simulink model "DrivingTestBench"  (R2026a)
settings: Solver=ode3  StartTime=0  StopTime=30  FixedStep=Ts  MaxStep=Ts
PreLoadFcn:
  | if(~configureDrivingTestBench.isdrivingApplicationOnPath())
  |     pathToDrivingApplication = fullfile(...
  |         matlabshared.supportpkg.getSupportPackageRoot,...
  |         "toolbox", "driving", "supportpackages", "variantgenerator", "drivingApplication");
  | 
  | 
  |     if (~exist("pathToDrivingApplication", "dir"))
  |         sldiagviewer.reportError(['This model requires you to download and install '...
  |             'Automated Driving Toolbox™ Test Suite for Euro NCAP® Protocols']);
  |     else
  |         addpath(fullfile(matlabshared.supportpkg.getSupportPackageRoot,"toolbox", "driving", "supportpackages", "variantgenerator", "drivingApplication"));
  |     end
  | end
values from neighbouring files (symbols this model uses):
  actorProfiles = repmat(actorProfile, 1, numActors)    [configureDrivingTestBench.m]
  BusActorPoses = Simulink.Bus    [configureDrivingTestBench.m]
  egoVehDyn = egoVehicleDynamicsParams(obj, egoInitialPose, actorProfiles(egoIndex))    [configureDrivingTestBench.m]
  m = worldActors(idx).actor_runtime.pose.matrix    [configureDrivingTestBench.m]
  maxAcc = 6    [configureDrivingTestBench.m]
  n = length(i)    [TargetBehavior.m]
  testStartPosition = [egoStartXPos egoStartYPos egoStartZPos]    [configureDrivingTestBench.m]
undefined symbols (not defined in the file or in its folder): aebEnable, cameraParams, Defined, driving, dtleThreshold, Ego, egoActorID, egoPathWidth, Lane, Left, lkaEnable, matlabshared, maxDecel, maxNumActors, Right, steadyStateSpeed, trackingParams, trackPosSelector, Ts, User
libraries: roadrunnerscenario x6, simulink_extras x6, drivingscenarioandsensors x4, trackingutilitieslib x1, drivinglib x1, simulink x1, autolibutils x1, autolibshared x1
(part 1 of 2)
settings Model: SILPILSystemUnderTest=refmodels  PauseTimes=16  SnapshotInterval=5  PacingRate=0.220000  Creator=The MathWorks, Inc.  LastModifiedBy=mraj
settings SolverCC: ZeroCrossAlgorithm=Adaptive  MinimalZcImpactIntegration=on
settings OptimizationCC: InlineInvariantSignals=on  SimCompilerOptimization=on
settings DebuggingCC: BusObjectLabelMismatch=none  PregeneratedLibrarySubsystemCodeDiagnostic=none  SubsystemReferenceDiagnosticForUnitTest=warning
settings ModelReferenceCC: CheckModelReferenceTargetMessage=none  EnableParallelModelReferenceBuilds=on  ModelReferenceNumInstancesAllowed=Single  PropagateVarSize=Only when enabling
settings RTWCC: SystemTargetFile=ert.tlc  GenerateReport=on  BuildConfiguration=Faster Runs  LaunchReport=on  LargeConstantGeneration=WriteOnlyDNNConstantsToDataFiles  Description=Embedded Coder
settings ERTTargetCC: DynamicArrayContainerType=coder::array  GenerateSampleERTMain=on
settings SimscapeCC: SimscapeNominalValues="[{\"value\":\"1\",\"unit\":\"A\"},{\"value\":\"1\",\"unit\":\"bar\"},{\"value\":\"1\",\"unit\":\"cm^2\"},{\"value\":\"1\",\"unit\":\"cm^3/s\"},{\"value\":\"1\",\"unit\":\"kJ/kg\"},{\"value\":\"1\",\"unit\":\"kW\"},{\"value\":\"1\",\"unit\":\"l\"},{\"value\":\"1\",\"unit\":\"N\"},{\"value\":\"1\",\"unit\":\"N*m\"},{\"value\":\"1\",\"unit\":\"V\"}]"  SimscapeLogType=none  SimscapeLogDataHistory=5000.0

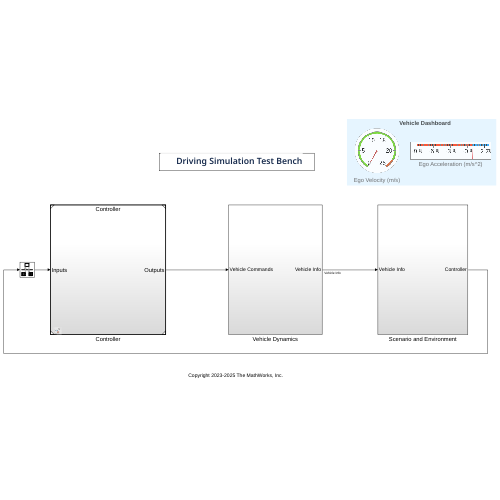
[thumbnail: Simulink's stored preview of the top-level diagram]
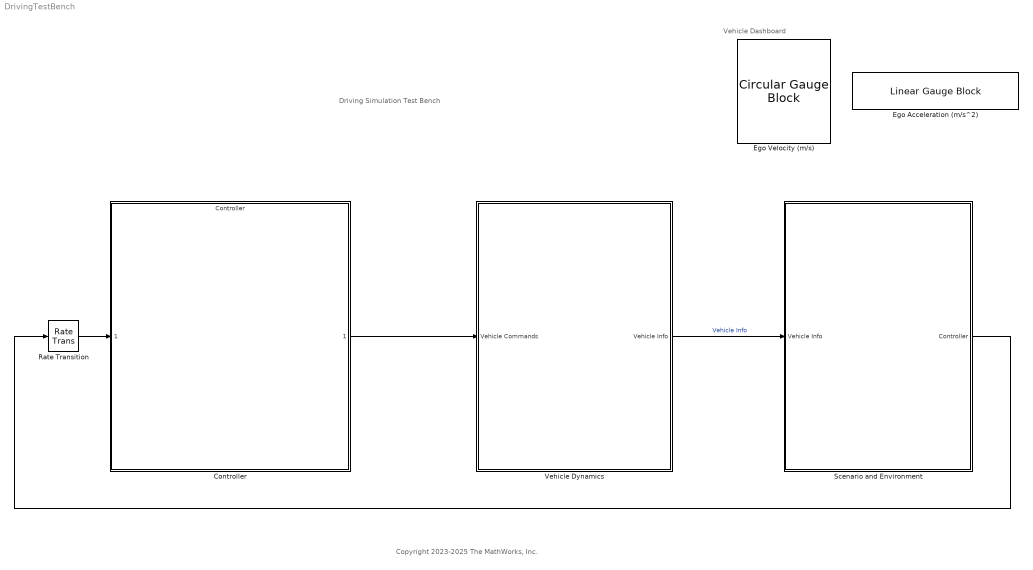
== system DrivingTestBench ==
  note: Copyright 2023-2025 The MathWorks, Inc.
  note: Driving Simulation Test Bench
  note: Vehicle Dashboard
  Controller : ModelReference  ModelNameDialog=Controller.slx  SimulationMode=Normal  CodeInterface=Top model  ModelReferenceVersion=12.11
  Ego Acceleration (m/s^2) : LinearGaugeBlock  LabelPosition=Hide  ScaleMin=-9.8  ScaleMax=3  TickInterval=3  FontColor=[0.0, 0.0, 0.0]
  Ego Velocity (m/s) : CircularGaugeBlock  LabelPosition=Hide  ScaleMax=25  FontColor=[0.0, 0.0, 0.0]
  Rate Transition : RateTransition  OutPortSampleTime=ControllerStepSize
  Scenario and Environment : Subsystem
  Vehicle Dynamics : Subsystem
  wires:
  Vehicle Dynamics/1(Vehicle Info) -> Scenario and Environment/1(Vehicle Info)  "Vehicle Info"
  Controller/1 -> Vehicle Dynamics/1(Vehicle Commands)
  Scenario and Environment/1(Controller) -> Rate Transition/1
  Rate Transition/1 -> Controller/1

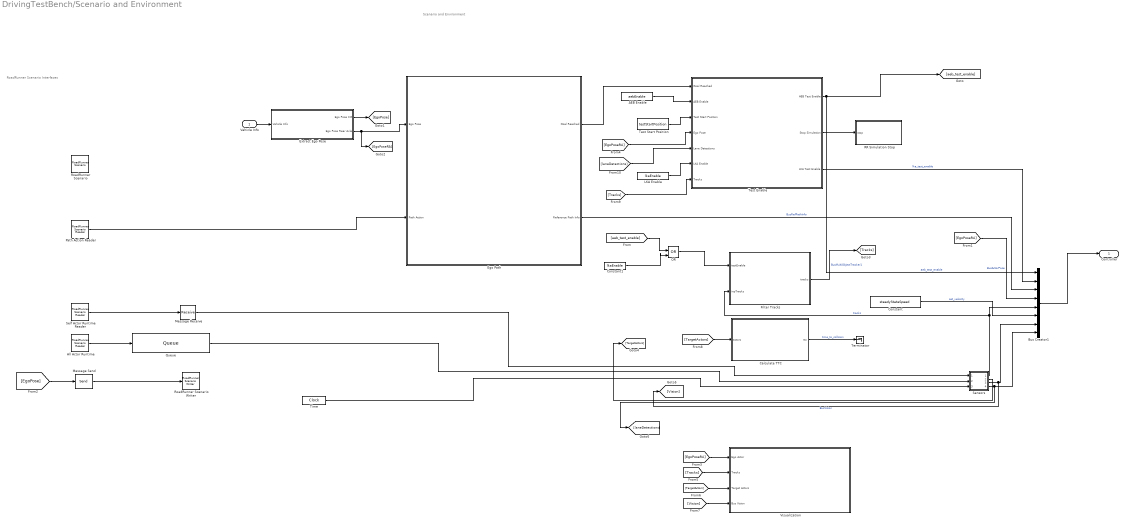
== system DrivingTestBench/Scenario and Environment ==
  note: RoadRunner Scenario Interfaces
  note: Scenario and Environment
  Vehicle Info : Inport
  AEB Enable : Constant  Value=aebEnable
  All Actor Runtime : roadrunnerscenario/RoadRunner Scenario Reader  TopicCategory=Actor  ActorCategory=All Types  ActionType=Path Following  EventType=User-Defined  TopicType=Actor Pose (Driving Scenario compatible)  VehicleType=Vehicle Specifications  TrafficSignalType=Traffic Signal Specifications  TrafficSignalControllerType=Traffic Signal Controller Specifications  UserDefinedAction=Action1  UserDefinedEvent=Event1  Filter=None  AdditionalRelationship=None  SensorTopic=Target Poses  LaneBoundaryOutputTopic=Ego-Lane  SensorID=1  SampleTime=Ts
  Bus Creator1 : BusCreator  Inputs=8  OutDataTypeStr=Bus: BusController
  Calculate TTC : MATLAB Function  TreatAsAtomicUnit=on  mask{actorProfiles=actorProfiles}
      mask prompts: actorProfiles "Actor Profiles"
  Constant : Constant  Value=steadyStateSpeed
  Constant1 : Constant  Value=lkaEnable
  Ego Path : Subsystem
      settings: PortSchema="{\"entries\":[{\"content\":{\"sides\":[{\"content\":{\"connectorIds\":[\"Out1\",\"Out2\"]},\"type\":\"ConnectorPlacement.EquallySpacedRectSide\",\"uuid\":\"4177219d-dfa9-425b-981e-5ad55aa9c50c\"},{\"content\":{\"connectorIds\":[\"In1\",\"In2\"],\"side\":\"RIGHT\"},\"type\":\"ConnectorPlacement.EquallySpacedRectSide\",\"uuid\":\"c7d91046-63f9-4309-950e-80e8e78c857b\"},{\"content\":{\"side\":\"TOP\"},\"type\":\"ConnectorPlacement.EquallySpacedRectSide\",\"uuid\":\"1ff1c131-cb31-4ea9-ae37-73c00ed985e9\"}]},\"type\":\"ConnectorPlacement.EquallySpacedConnector\",\"uuid\":\"26604a6c-d9bc-4865-baff-6ddacb0afb6e\"}],\"packageUris\":[\"http://schema.mathworks.com/mf0/Connector/R2020b\"],\"version\":\"1.0\"}"
  Extract Ego Pose : Subsystem
  Filter Tracks : MATLAB Function  TreatAsAtomicUnit=on
  LKA Enable : Constant  Value=lkaEnable
  Message Receive : Receive  InputPortMessageModes=m  SampleTime=Ts
  Message Send : Send  OutputPortMessageModes=m
  OR : Logic  Operator=OR  IconShape=distinctive  AllPortsSameDT=off  OutDataTypeStr=boolean
  Path Action Reader : roadrunnerscenario/RoadRunner Scenario Reader  TopicCategory=Action  ActorCategory=All Types  ActionType=Path Following  EventType=User-Defined  TopicType=Actor Specifications  VehicleType=Vehicle Specifications  TrafficSignalType=Traffic Signal Specifications  TrafficSignalControllerType=Traffic Signal Controller Specifications  UserDefinedAction=Action1  UserDefinedEvent=Event1  Filter=Self  AdditionalRelationship=None  SensorTopic=Target Poses  LaneBoundaryOutputTopic=Ego-Lane  SensorID=1  SampleTime=Ts
  Queue : Queue  InputPortMessageModes=m  OutputPortMessageModes=m  OverwriteOldest=on  Capacity=maxNumActors+1
  RR Simulation Stop : MATLAB Function  TreatAsAtomicUnit=on
  RoadRunner Scenario : roadrunnerscenario/RoadRunner Scenario  ScenarioFileName=auto  ActorIDLinkedToModel=1  SampleTime=0.02  OpenRoadRunnerAtSimulationStart=on  EnableSimulationLoggingInRoadRunner=off  UserDefinedActions={}  UserDefinedEvents={}  PathPoints=500
  RoadRunner Scenario Writer : roadrunnerscenario/RoadRunner Scenario Writer  TopicCategory=Actor  ActorCategory=All Types  EventType=Action Complete  UserDefinedEvent=Event1  VehicleType=Vehicle Pose  TopicType=Actor Pose
  Self Actor Runtime Reader : roadrunnerscenario/RoadRunner Scenario Reader  TopicCategory=Actor  ActorCategory=All Types  ActionType=Path Following  EventType=User-Defined  TopicType=Actor Pose (Driving Scenario compatible)  VehicleType=Vehicle Specifications  TrafficSignalType=Traffic Signal Specifications  TrafficSignalControllerType=Traffic Signal Controller Specifications  UserDefinedAction=Action1  UserDefinedEvent=Event1  Filter=Self  AdditionalRelationship=None  SensorTopic=Target Poses  LaneBoundaryOutputTopic=Ego-Lane  SensorID=1  SampleTime=Ts
  Sensors : Subsystem
  Terminator : Terminator
  Test Enable : Subsystem
  Test Start Position : Constant  Value=testStartPosition
  Time : DigitalClock  SampleTime=Ts
  Visualization : Subsystem
  Controller : Outport  OutDataTypeStr=Bus: BusController
  wires:
  Self Actor Runtime Reader/1 -> Message Receive/1
  All Actor Runtime/1 -> Queue/1
  Vehicle Info/1 -> Extract Ego Pose/1(Vehicle Info)
  Message Send/1 -> RoadRunner Scenario Writer/1
  Ego Path/2(Goal Reached) -> Test Enable/1(Goal Reached)
  AEB Enable/1 -> Test Enable/2(AEB Enable)
  Test Start Position/1 -> Test Enable/3(Test Start Position)
  Test Enable/2(Stop Simulation) -> RR Simulation Stop/1(stop)
  Path Action Reader/1 -> Ego Path/1(Path Action)
  OR/1 -> Filter Tracks/1(testEnable)
  Filter Tracks/1(tracks) -> [Tracks]  "BusMultiObjectTracker1"
  Extract Ego Pose/1(Ego Pose CG) -> [EgoPose]
  [EgoPoseRA] -> Test Enable/4(Ego Pose)
  [EgoPose] -> Message Send/1
  Extract Ego Pose/2(Ego Pose Rear Axle) -> Ego Path/2(Ego Pose), [EgoPoseRA]
  [EgoPoseRA] -> Visualization/1(Ego Actor)
  [Tracks] -> Visualization/2(Tracks)
  [TargetActors] -> Visualization/3(Target Actors)
  [Vision] -> Visualization/4(Bus Vision)
  Calculate TTC/1(ttc) -> Terminator/1  "time_to_collision"
  [TargetActors] -> Calculate TTC/1(actors)
  [Tracks] -> Test Enable/7(Tracks)
  [laneDetections] -> Test Enable/5(Lane Detections)
  LKA Enable/1 -> Test Enable/6(LKA Enable)
  [aeb_test_enable] -> OR/1
  Constant1/1 -> OR/2
  Sensors/4(Lane Detections) -> [laneDetections], Bus Creator1/8
  Test Enable/3(LKA Test Enable) -> Bus Creator1/2  "lka_test_enable"
  Bus Creator1/1 -> Controller/1
  Sensors/3(Vision) -> [Vision], Bus Creator1/7  "BusVision"
  Constant/1 -> Bus Creator1/6  "set_velocity"
  Ego Path/1(Reference Path Info) -> Bus Creator1/3  "BusRefPathInfo"
  [EgoPoseRA] -> Bus Creator1/4  "BusActorPose"
  Time/1 -> Sensors/3(System Time)
  Sensors/2(Actors) -> [TargetActors]
  Queue/1 -> Sensors/2(All Actors)
  Sensors/1(Tracks) -> Filter Tracks/2(inpTracks), Bus Creator1/5  "tracks"
  Test Enable/1(AEB Test Enable) -> [aeb_test_enable], Bus Creator1/1  "aeb_test_enable"
  Message Receive/1 -> Sensors/1(Bus Actor Pose)

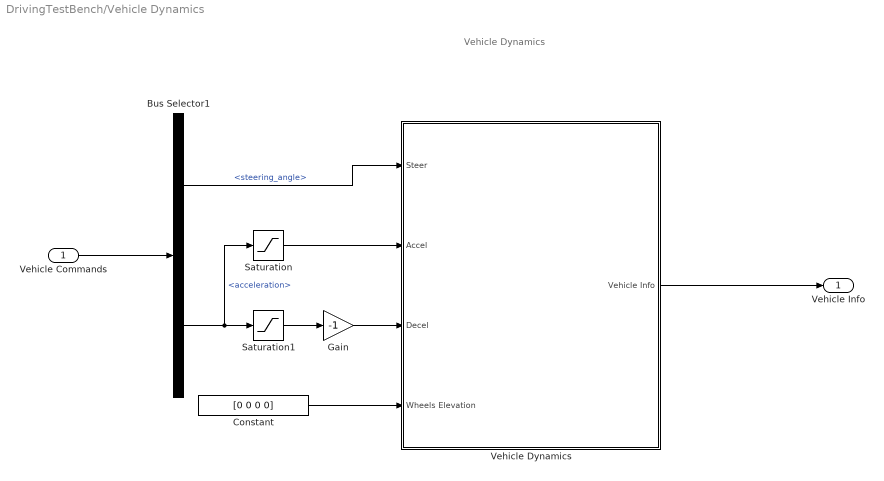
== system DrivingTestBench/Vehicle Dynamics ==
  note: Vehicle Dynamics
  Vehicle Commands : Inport
  Bus Selector1 : BusSelector  OutputSignals=steering_angle,acceleration
  Constant : Constant  Value=[0 0 0 0]  SampleTime=Ts
  Gain : Gain  Gain=-1
  Saturation : Saturate  UpperLimit=maxAcc  LowerLimit=0
  Saturation1 : Saturate  UpperLimit=0  LowerLimit=maxDecel
  Vehicle Dynamics : Subsystem  Variant=on
  Vehicle Info : Outport  VectorParamsAs1DForOutWhenUnconnected=off
  wires:
  Saturation1/1 -> Gain/1
  Bus Selector1/1 -> Vehicle Dynamics/1(Steer)  "<steering_angle>"
  Bus Selector1/2 -> Saturation/1, Saturation1/1  "<acceleration>"
  Vehicle Commands/1 -> Bus Selector1/1
  Saturation/1 -> Vehicle Dynamics/2(Accel)
  Gain/1 -> Vehicle Dynamics/3(Decel)
  Constant/1 -> Vehicle Dynamics/4(Wheels Elevation)
  Vehicle Dynamics/1(Vehicle Info) -> Vehicle Info/1

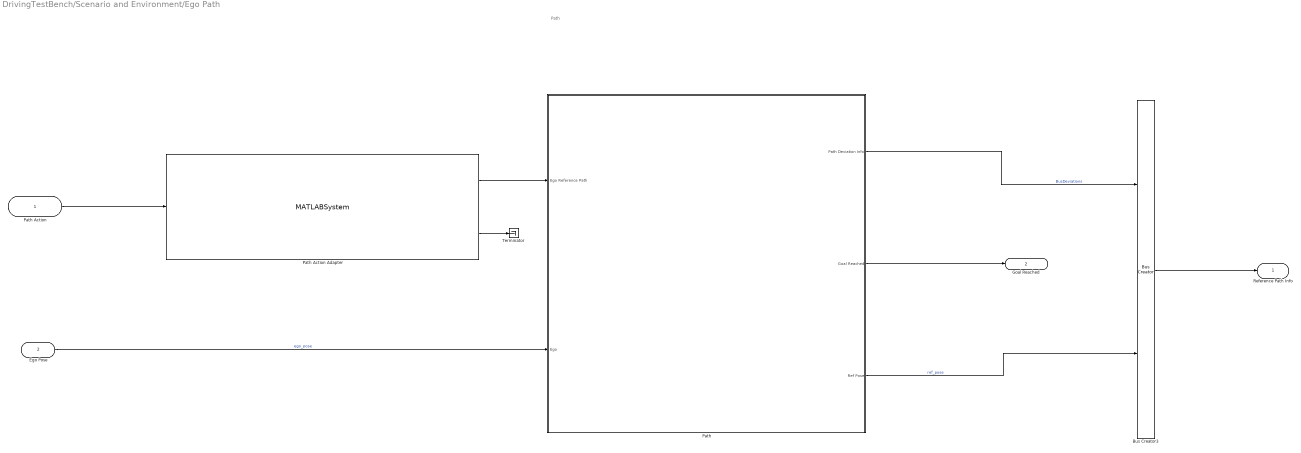
== system DrivingTestBench/Scenario and Environment/Ego Path ==
  note: Path
  Path Action : Inport  SampleTime=Ts
  Ego Pose : Inport  Port=2
  Bus Creator3 : BusCreator  Inputs=2
  Path : Subsystem
  Path Action Adapter : MATLABSystem  InputPortMessageModes=m  System=drivingApplication.internal.path.PathActionAdapter  SpaceResolution=discretizationDistance  MaxNumPoints=refPathSize
      mask Type: drivingApplication.internal.path.PathActionAdapter
  Terminator : Terminator
  Reference Path Info : Outport
  Goal Reached : Outport  Port=2
  wires:
  Path/2(Goal Reached) -> Goal Reached/1
  Ego Pose/1 -> Path/2(Ego)  "ego_pose"
  Path Action Adapter/1 -> Path/1(Ego Reference Path)
  Path Action Adapter/2 -> Terminator/1
  Bus Creator3/1 -> Reference Path Info/1
  Path/1(Path Deviation Info) -> Bus Creator3/1  "BusDeviations"
  Path/3(Ref Pose) -> Bus Creator3/2  "ref_pose"
  Path Action/1 -> Path Action Adapter/1

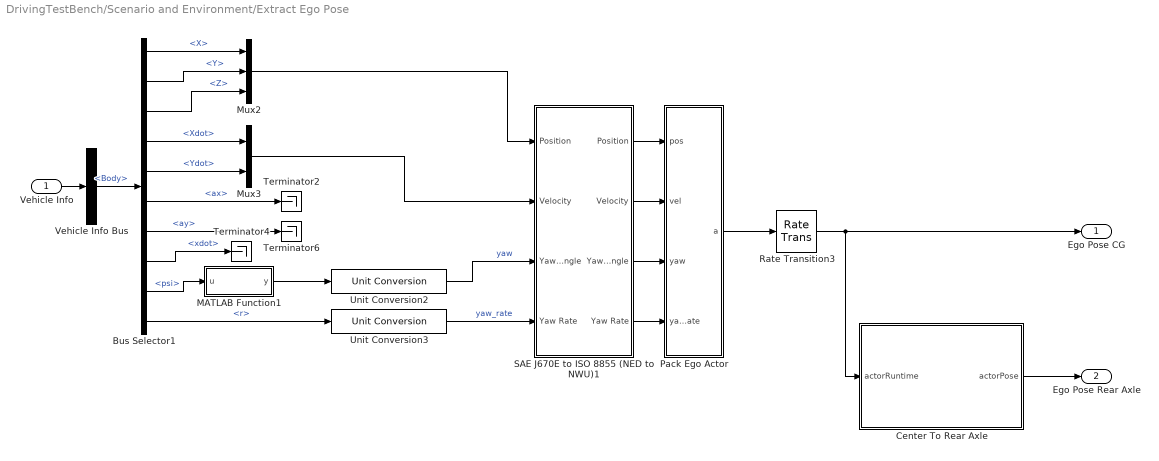
== system DrivingTestBench/Scenario and Environment/Extract Ego Pose ==
  Vehicle Info : Inport
  Bus Selector1 : BusSelector  OutputSignals=InertFrm.Cg.Disp.X,InertFrm.Cg.Disp.Y,InertFrm.Cg.Disp.Z,InertFrm.Cg.Vel.Xdot,InertFrm.Cg.Vel.Ydot,BdyFrm.Cg.Acc.ax,BdyFrm.Cg.Acc.ay,BdyFrm.Cg.Vel.xdot,InertFrm.Cg.Ang.psi,BdyFrm.Cg.AngVel.r
  Center To Rear Axle : MATLAB Function  TreatAsAtomicUnit=on  mask{CGToRearAxle=egoVehDyn.CGToRearAxle}
      mask prompts: CGToRearAxle "Center to rear axle offset"
  MATLAB Function1 : MATLAB Function  TreatAsAtomicUnit=on
  Mux2 : Mux  Inputs=3
  Mux3 : Mux  Inputs=2
  Pack Ego Actor : MATLAB Function  TreatAsAtomicUnit=on  mask{egoActorID=egoActorID}
      mask prompts: egoActorID "Ego Actor ID"
  Rate Transition3 : RateTransition  OutPortSampleTime=Ts
  SAE J670E to ISO 8855 (NED to NWU)1 : Subsystem
  Terminator2 : Terminator
  Terminator4 : Terminator
  Terminator6 : Terminator
  Unit Conversion2 : UnitConversion  OutputType=Inherit: Inherit via back propagation
  Unit Conversion3 : UnitConversion  OutputType=Inherit: Inherit via back propagation
  Vehicle Info Bus : BusSelector  OutputSignals=Body
  Ego Pose CG : Outport
  Ego Pose Rear Axle : Outport  Port=2  SampleTime=Ts
  wires:
  Vehicle Info Bus/1 -> Bus Selector1/1  "<Body>"
  Rate Transition3/1 -> Center To Rear Axle/1(actorRuntime), Ego Pose CG/1
  Vehicle Info/1 -> Vehicle Info Bus/1
  Pack Ego Actor/1(a) -> Rate Transition3/1
  SAE J670E to ISO 8855 (NED to NWU)1/1("Position ") -> Pack Ego Actor/1(pos)
  SAE J670E to ISO 8855 (NED to NWU)1/2("Velocity ") -> Pack Ego Actor/2(vel)
  SAE J670E to ISO 8855 (NED to NWU)1/3("Yaw Angle ") -> Pack Ego Actor/3(yaw)
  SAE J670E to ISO 8855 (NED to NWU)1/4("Yaw Rate ") -> Pack Ego Actor/4(yawRate)
  MATLAB Function1/1(y) -> Unit Conversion2/1
  Unit Conversion2/1 -> SAE J670E to ISO 8855 (NED to NWU)1/3(Yaw Angle)  "yaw"
  Unit Conversion3/1 -> SAE J670E to ISO 8855 (NED to NWU)1/4(Yaw Rate)  "yaw_rate"
  Bus Selector1/10 -> Unit Conversion3/1  "<r>"
  Bus Selector1/9 -> MATLAB Function1/1(u)  "<psi>"
  Bus Selector1/8 -> Terminator4/1  "<xdot>"
  Bus Selector1/7 -> Terminator6/1  "<ay>"
  Bus Selector1/6 -> Terminator2/1  "<ax>"
  Bus Selector1/5 -> Mux3/2  "<Ydot>"
  Bus Selector1/4 -> Mux3/1  "<Xdot>"
  Bus Selector1/2 -> Mux2/2  "<Y>"
  Bus Selector1/1 -> Mux2/1  "<X>"
  Mux2/1 -> SAE J670E to ISO 8855 (NED to NWU)1/1(Position)
  Mux3/1 -> SAE J670E to ISO 8855 (NED to NWU)1/2(Velocity)
  Bus Selector1/3 -> Mux2/3  "<Z>"
  Center To Rear Axle/1(actorPose) -> Ego Pose Rear Axle/1

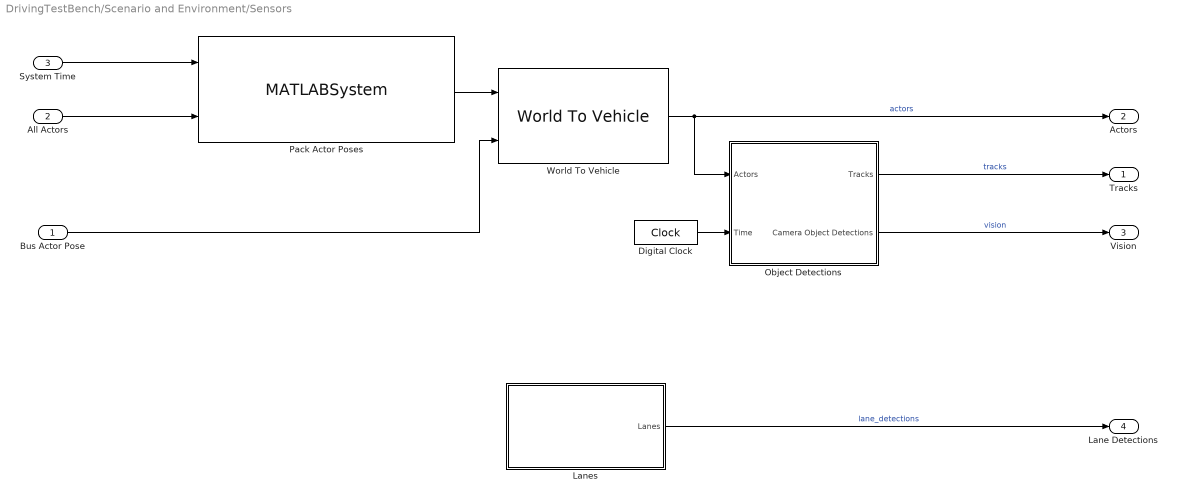
== system DrivingTestBench/Scenario and Environment/Sensors ==
  Bus Actor Pose : Inport
  All Actors : Inport  Port=2
  System Time : Inport  Port=3
  Digital Clock : DigitalClock  SampleTime=Ts
  Lanes : Subsystem  Variant=on  VariantControlMode=label  LabelModeActiveChoice=No Lanes
  Object Detections : Subsystem  Variant=on  VariantControlMode=label  LabelModeActiveChoice=allSensors
  Pack Actor Poses : MATLABSystem  InputPortMessageModes=n,m  System=drivingApplication.internal.utils.PackTargetActorPoses  EgoActorID=egoActorID  ActorProfiles=actorProfiles  DefaultActorPoses="Simulink.Bus.createMATLABStruct(\"BusActorPoses\")"
      mask Type: drivingApplication.internal.utils.PackTargetActorPoses
  World To Vehicle : drivingscenarioandsensors/World To Vehicle  BusNameSource=Auto  BusName=BusActors  SimulateUsing=Interpreted execution
  Tracks : Outport
  Actors : Outport  Port=2
  Vision : Outport  Port=3  OutDataTypeStr=Bus: BusVision
  Lane Detections : Outport  Port=4  OutDataTypeStr=Bus: LaneBus
  wires:
  All Actors/1 -> Pack Actor Poses/2
  Object Detections/1(Tracks) -> Tracks/1  "tracks"
  World To Vehicle/1 -> Object Detections/1(Actors), Actors/1  "actors"
  System Time/1 -> Pack Actor Poses/1
  Pack Actor Poses/1 -> World To Vehicle/1
  Bus Actor Pose/1 -> World To Vehicle/2
  Lanes/1(Lanes) -> Lane Detections/1  "lane_detections"
  Digital Clock/1 -> Object Detections/2(Time)
  Object Detections/2(Camera Object Detections) -> Vision/1  "vision"

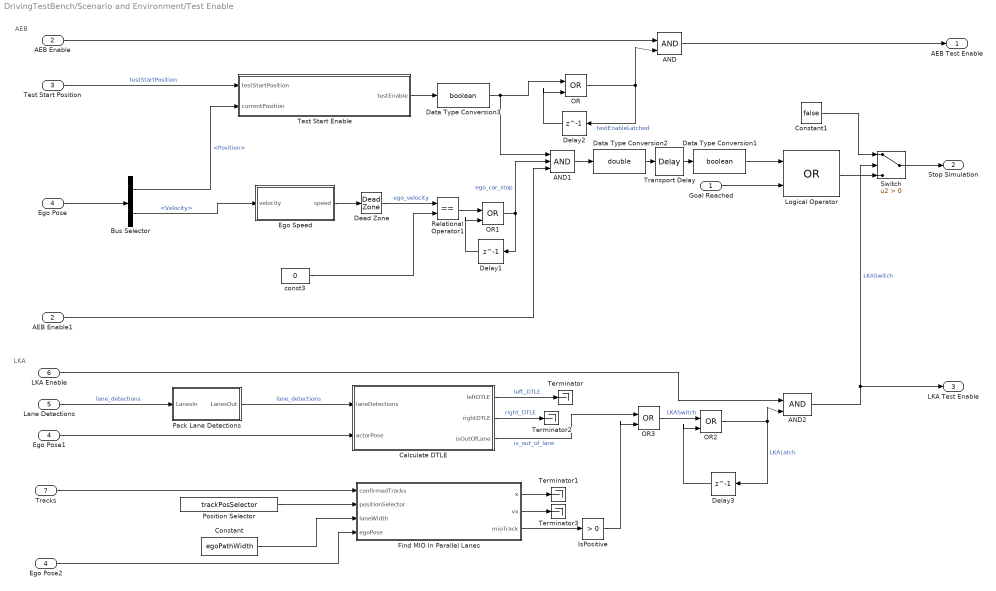
== system DrivingTestBench/Scenario and Environment/Test Enable ==
  note: LKA
  note: AEB
  Goal Reached : Inport
  AEB Enable : Inport  Port=2
  Test Start Position : Inport  Port=3
  Ego Pose : Inport  Port=4
  Lane Detections : Inport  Port=5
  LKA Enable : Inport  Port=6
  Tracks : Inport  Port=7
  AEB Enable1 : InportShadow  Port=2
  AND : Logic  IconShape=distinctive  AllPortsSameDT=off  OutDataTypeStr=boolean
  AND1 : Logic  Inputs=3  IconShape=distinctive  AllPortsSameDT=off  OutDataTypeStr=boolean
  AND2 : Logic  IconShape=distinctive  AllPortsSameDT=off  OutDataTypeStr=boolean
  Bus Selector : BusSelector  OutputSignals=Position,Velocity
  Calculate DTLE : MATLAB Function  TreatAsAtomicUnit=on  mask{actorProfiles=actorProfiles, DTLEThreshold=dtleThreshold, egoActorID=egoActorID}
      mask prompts: actorProfiles "Actor Profiles"; DTLEThreshold "DTLE Threshold"; egoActorID "Ego Actor ID"
  Constant : Constant  Value=egoPathWidth
  Constant1 : Constant  Value=false  OutDataTypeStr=boolean
  Data Type Conversion1 : DataTypeConversion  OutDataTypeStr=boolean  SaturateOnIntegerOverflow=off  RndMeth=Floor
  Data Type Conversion2 : DataTypeConversion  OutDataTypeStr=double  SaturateOnIntegerOverflow=off  RndMeth=Floor
  Data Type Conversion3 : DataTypeConversion  OutDataTypeStr=boolean  SaturateOnIntegerOverflow=off  RndMeth=Floor
  Dead Zone : DeadZone  LowerValue=-inf  UpperValue=0.001
  Delay1 : Delay  DelayLength=1
  Delay2 : Delay  DelayLength=1
  Delay3 : Delay  DelayLength=1
  Ego Pose1 : InportShadow  Port=4
  Ego Pose2 : InportShadow  Port=4
  Ego Speed : MATLAB Function  TreatAsAtomicUnit=on
  Find MIO In Parallel Lanes : MATLAB Function  TreatAsAtomicUnit=on
  IsPositive : simulink/Logic and Bit Operations/Compare To Zero  relop=>  OutDataTypeStr=boolean
  Logical Operator : Logic  Operator=OR  AllPortsSameDT=off  OutDataTypeStr=boolean
  OR{,1..3} (4 alike) : Logic  Operator=OR  IconShape=distinctive  AllPortsSameDT=off  OutDataTypeStr=boolean
  Pack Lane Detections : Subsystem
  Position Selector : Constant  Value=trackPosSelector
  Relational Operator1 : RelationalOperator  Operator===  OutDataTypeStr=boolean  RndMeth=Simplest  InputSameDT=off
  Switch : Switch  Criteria=u2 > Threshold  SaturateOnIntegerOverflow=off  InputSameDT=off
  Terminator{,1..3} (4 alike) : Terminator
  Test Start Enable : MATLAB Function  TreatAsAtomicUnit=on
  Transport Delay : TransportDelay  DelayTime=2  BufferSize=7000
  const3 : Constant  Value=0  SampleTime=-1
  AEB Test Enable : Outport
  Stop Simulation : Outport  Port=2
  LKA Test Enable : Outport  Port=3
  wires:
  Test Start Position/1 -> Test Start Enable/1(testStartPosition)  "testStartPosition"
  AEB Enable/1 -> AND/1
  AND/1 -> AEB Test Enable/1
  Goal Reached/1 -> Logical Operator/2
  Test Start Enable/1(testEnable) -> Data Type Conversion3/1
  Ego Speed/1(speed) -> Dead Zone/1
  Bus Selector/2 -> Ego Speed/1(velocity)  "<Velocity>"
  AEB Enable1/1 -> AND1/3
  AND1/1 -> Data Type Conversion2/1
  Data Type Conversion1/1 -> Logical Operator/1
  Transport Delay/1 -> Data Type Conversion1/1
  Data Type Conversion2/1 -> Transport Delay/1
  Logical Operator/1 -> Switch/3
  const3/1 -> Relational Operator1/2
  Bus Selector/1 -> Test Start Enable/2(currentPosition)  "<Position>"
  Data Type Conversion3/1 -> OR/1, AND1/1
  Delay2/1 -> OR/2
  OR/1 -> AND/2, Delay2/1  "testEnableLatched"
  Dead Zone/1 -> Relational Operator1/1  "ego_velocity"
  OR1/1 -> AND1/2, Delay1/1  "ego_car_stop"
  Delay1/1 -> OR1/2
  Relational Operator1/1 -> OR1/1
  Ego Pose/1 -> Bus Selector/1
  Calculate DTLE/3(isOutOfLane) -> OR3/1  "is_out_of_lane"
  Ego Pose1/1 -> Calculate DTLE/2(actorPose)
  OR3/1 -> OR2/1  "LKASwitch"
  Calculate DTLE/1(leftDTLE) -> Terminator/1  "left_DTLE"
  OR2/1 -> Delay3/1, AND2/2  "LKALatch"
  Calculate DTLE/2(rightDTLE) -> Terminator2/1  "right_DTLE"
  Lane Detections/1 -> Pack Lane Detections/1(LanesIn)  "lane_detections"
  Delay3/1 -> OR2/2
  Pack Lane Detections/1(LanesOut) -> Calculate DTLE/1(laneDetections)  "lane_detections"
  Tracks/1 -> Find MIO In Parallel Lanes/1(confirmedTracks)
  Position Selector/1 -> Find MIO In Parallel Lanes/2(positionSelector)
  Constant/1 -> Find MIO In Parallel Lanes/3(laneWidth)
  Ego Pose2/1 -> Find MIO In Parallel Lanes/4(egoPose)
  Find MIO In Parallel Lanes/1(x) -> Terminator1/1
  Find MIO In Parallel Lanes/2(vx) -> Terminator3/1
  Find MIO In Parallel Lanes/3(mioTrack) -> IsPositive/1
  IsPositive/1 -> OR3/2
  Switch/1 -> Stop Simulation/1
  Constant1/1 -> Switch/1
  AND2/1 -> LKA Test Enable/1, Switch/2  "LKASwitch"
  LKA Enable/1 -> AND2/1

== system DrivingTestBench/Scenario and Environment/Visualization ==
  Ego Actor : Inport  SampleTime=Ts
  Tracks : Inport  Port=2  SampleTime=Ts
  Target Actors : Inport  Port=3
  Bus Vision : Inport  Port=4  SampleTime=Ts
  Plot Run Time Results : MATLABSystem  System=PlotRunTimeResults  Camera=cameraParams  Radar=radarParams  EgoCarID=egoActorID  ActorProfiles=actorProfiles  IsDisplayEnabled=off  SampleTime=0.03
      mask Type: PlotRunTimeResults
  wires:
  Target Actors/1 -> Plot Run Time Results/1
  Tracks/1 -> Plot Run Time Results/3
  Bus Vision/1 -> Plot Run Time Results/4
  Ego Actor/1 -> Plot Run Time Results/2

== system DrivingTestBench/Vehicle Dynamics/Vehicle Dynamics ==
  Steer : Inport
  Accel : Inport  Port=2
  Decel : Inport  Port=3
  Wheels Elevation : Inport  Port=4
  14DOF : Subsystem  VariantControl="vehicle == \"14DOF\""
  3DOF : Subsystem  VariantControl="vehicle == \"3DOF\""
  Vehicle Info : Outport

== system DrivingTestBench/Scenario and Environment/Ego Path/Path ==
  note: Path
  Ego Reference Path : Inport
  Ego : Inport  Port=2
  Bus Creator : BusCreator  Inputs=3  OutDataTypeStr=Bus: BusDeviations
      settings: InheritFromInputs=off
  Ego Reference Path Predictor : MATLABSystem  System=drivingApplication.internal.path.ActorPosePredictor  PredictionHorizon=predictionHorizon  DistanceFromCGToRear=egoVehDyn.CGToRearAxle  SampleTime=Ts
      mask Type: drivingApplication.internal.path.ActorPosePredictor
  Path Deviation Info : Outport  OutDataTypeStr=Bus: BusDeviations
  Goal Reached : Outport  Port=2
  Ref Pose : Outport  Port=3
  wires:
  Ego Reference Path Predictor/1 -> Bus Creator/1
  Ego/1 -> Ego Reference Path Predictor/1
  Ego Reference Path/1 -> Ego Reference Path Predictor/2
  Ego Reference Path Predictor/2 -> Bus Creator/2  "lateral_deviation"
  Ego Reference Path Predictor/3 -> Bus Creator/3
  Bus Creator/1 -> Path Deviation Info/1
  Ego Reference Path Predictor/4 -> Goal Reached/1
  Ego Reference Path Predictor/5 -> Ref Pose/1

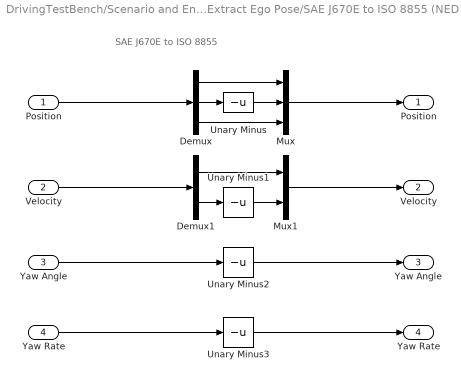
== system DrivingTestBench/Scenario and Environment/Extract Ego Pose/SAE J670E to ISO 8855 (NED to NWU)1 ==
  note: SAE J670E to ISO 8855
  Position : Inport  Unit=m
  Velocity : Inport  Port=2  Unit=m/s
  Yaw Angle : Inport  Port=3  Unit=deg
  Yaw Rate : Inport  Port=4  Unit=deg/s
  Demux : Demux  Outputs=3
  Demux1 : Demux  Outputs=2
  Mux : Mux  Inputs=3
  Mux1 : Mux  Inputs=2
  Unary Minus{,1..3} (4 alike) : UnaryMinus
  "Position " : Outport  VectorParamsAs1DForOutWhenUnconnected=off
  "Velocity " : Outport  Port=2  VectorParamsAs1DForOutWhenUnconnected=off
  "Yaw Angle " : Outport  Port=3  VectorParamsAs1DForOutWhenUnconnected=off
  "Yaw Rate " : Outport  Port=4  VectorParamsAs1DForOutWhenUnconnected=off
  wires:
  Unary Minus3/1 -> "Yaw Rate "/1
  Unary Minus2/1 -> "Yaw Angle "/1
  Velocity/1 -> Demux1/1
  Position/1 -> Demux/1
  Mux/1 -> "Position "/1
  Mux1/1 -> "Velocity "/1
  Demux1/1 -> Mux1/1
  Demux1/2 -> Unary Minus1/1
  Unary Minus1/1 -> Mux1/2
  Unary Minus/1 -> Mux/2
  Demux/2 -> Unary Minus/1
  Demux/1 -> Mux/1
  Yaw Angle/1 -> Unary Minus2/1
  Yaw Rate/1 -> Unary Minus3/1
  Demux/3 -> Mux/3

== system DrivingTestBench/Scenario and Environment/Sensors/Lanes ==
  note: Lane Sensors
  No Lanes : Subsystem  VariantControl=No Lanes
  Vision : Subsystem  VariantControl=Vision
  Lanes : Outport  OutDataTypeStr=Bus: LaneBus

== system DrivingTestBench/Scenario and Environment/Sensors/Object Detections ==
  note: Sensors
  Actors : Inport
  Time : Inport  Port=2
  Camera and Radar : Subsystem  VariantControl=allSensors
  Ground Truth : Subsystem  VariantControl=groundTruth
  Tracks : Outport
  Camera Object Detections : Outport  Port=2

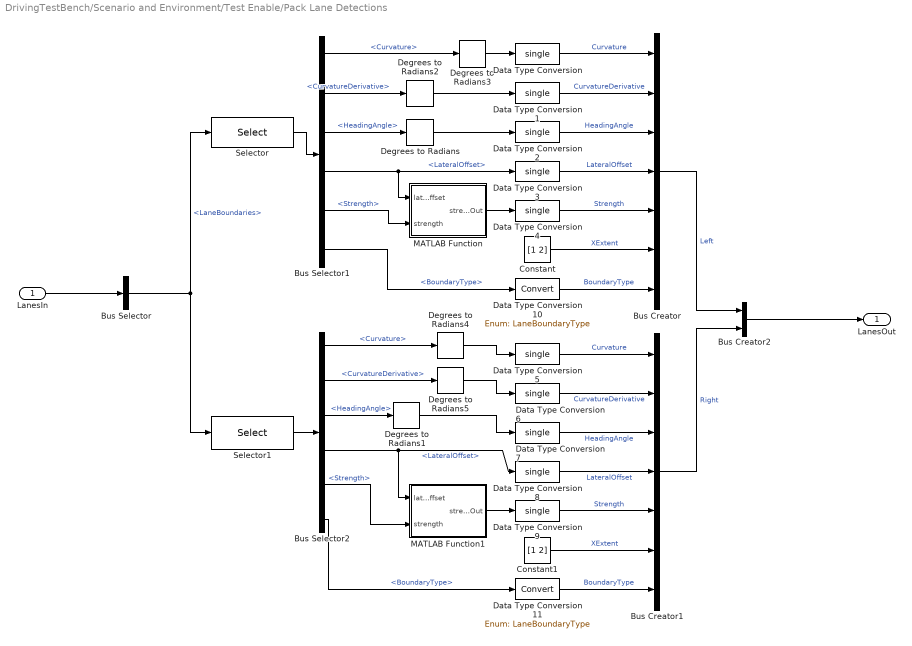
== system DrivingTestBench/Scenario and Environment/Test Enable/Pack Lane Detections ==
  LanesIn : Inport
  Bus Creator : BusCreator  Inputs=7  OutDataTypeStr=Bus: LaneSensorBoundaries
  Bus Creator1 : BusCreator  Inputs=7  OutDataTypeStr=Bus: LaneSensorBoundaries
  Bus Creator2 : BusCreator  Inputs=Left,Right  OutDataTypeStr=Bus: LaneSensor
  Bus Selector : BusSelector  OutputSignals=LaneBoundaries
  Bus Selector1 : BusSelector  OutputSignals=Curvature,CurvatureDerivative,HeadingAngle,LateralOffset,Strength,BoundaryType
  Bus Selector2 : BusSelector  OutputSignals=Curvature,CurvatureDerivative,HeadingAngle,LateralOffset,Strength,BoundaryType
  Constant : Constant  Value=[1 2]  OutDataTypeStr=single
  Constant1 : Constant  Value=[1 2]  OutDataTypeStr=single
  Data Type Conversion{,1..9} (10 alike) : DataTypeConversion  OutDataTypeStr=single  SaturateOnIntegerOverflow=off  RndMeth=Floor
  Data Type Conversion10 : DataTypeConversion  OutDataTypeStr=Enum: LaneBoundaryType  SaturateOnIntegerOverflow=off  RndMeth=Floor
  Data Type Conversion11 : DataTypeConversion  OutDataTypeStr=Enum: LaneBoundaryType  SaturateOnIntegerOverflow=off  RndMeth=Floor
  Degrees to Radians{,1..5} (6 alike) : simulink_extras/Transformations/Degrees to Radians
  MATLAB Function : MATLAB Function  TreatAsAtomicUnit=on
  MATLAB Function1 : MATLAB Function  TreatAsAtomicUnit=on
  Selector : Selector  InputPortWidth=2  IndexOptions=Index vector (dialog)  Indices=1  OutputSizes=1  RuntimeRangeChecks=on
  Selector1 : Selector  InputPortWidth=2  IndexOptions=Index vector (dialog)  Indices=2  OutputSizes=1
  LanesOut : Outport  VectorParamsAs1DForOutWhenUnconnected=off
  wires:
  LanesIn/1 -> Bus Selector/1
  Bus Selector/1 -> Selector/1, Selector1/1  "<LaneBoundaries>"
  Selector/1 -> Bus Selector1/1
  Bus Selector1/2 -> Degrees to Radians2/1  "<CurvatureDerivative>"
  Bus Selector1/1 -> Degrees to Radians3/1  "<Curvature>"
  Bus Selector1/3 -> Degrees to Radians/1  "<HeadingAngle>"
  Bus Selector1/4 -> Data Type Conversion3/1, MATLAB Function/1(laterOffset)  "<LateralOffset>"
  Data Type Conversion/1 -> Bus Creator/1  "Curvature"
  Data Type Conversion1/1 -> Bus Creator/2  "CurvatureDerivative"
  Data Type Conversion2/1 -> Bus Creator/3  "HeadingAngle"
  Data Type Conversion3/1 -> Bus Creator/4  "LateralOffset"
  Data Type Conversion4/1 -> Bus Creator/5  "Strength"
  Data Type Conversion9/1 -> Bus Creator1/5  "Strength"
  Data Type Conversion6/1 -> Bus Creator1/2  "CurvatureDerivative"
  Data Type Conversion7/1 -> Bus Creator1/3  "HeadingAngle"
  Data Type Conversion8/1 -> Bus Creator1/4  "LateralOffset"
  Data Type Conversion5/1 -> Bus Creator1/1  "Curvature"
  Bus Selector2/1 -> Degrees to Radians4/1  "<Curvature>"
  Selector1/1 -> Bus Selector2/1
  Bus Selector2/4 -> MATLAB Function1/1(laterOffset), Data Type Conversion8/1  "<LateralOffset>"
  Bus Selector2/2 -> Degrees to Radians5/1  "<CurvatureDerivative>"
  Bus Selector2/3 -> Degrees to Radians1/1  "<HeadingAngle>"
  Bus Creator2/1 -> LanesOut/1
  Bus Creator/1 -> Bus Creator2/1  "Left"
  Bus Creator1/1 -> Bus Creator2/2  "Right"
  Constant/1 -> Bus Creator/6  "XExtent"
  Bus Selector1/6 -> Data Type Conversion10/1  "<BoundaryType>"
  Bus Selector2/6 -> Data Type Conversion11/1  "<BoundaryType>"
  Constant1/1 -> Bus Creator1/6  "XExtent"
  Data Type Conversion10/1 -> Bus Creator/7  "BoundaryType"
  Data Type Conversion11/1 -> Bus Creator1/7  "BoundaryType"
  MATLAB Function/1(strengthOut) -> Data Type Conversion4/1
  Bus Selector1/5 -> MATLAB Function/2(strength)  "<Strength>"
  MATLAB Function1/1(strengthOut) -> Data Type Conversion9/1
  Bus Selector2/5 -> MATLAB Function1/2(strength)  "<Strength>"
  Degrees to Radians1/1 -> Data Type Conversion7/1
  Degrees to Radians4/1 -> Data Type Conversion5/1
  Degrees to Radians5/1 -> Data Type Conversion6/1
  Degrees to Radians3/1 -> Data Type Conversion/1
  Degrees to Radians2/1 -> Data Type Conversion1/1
  Degrees to Radians/1 -> Data Type Conversion2/1

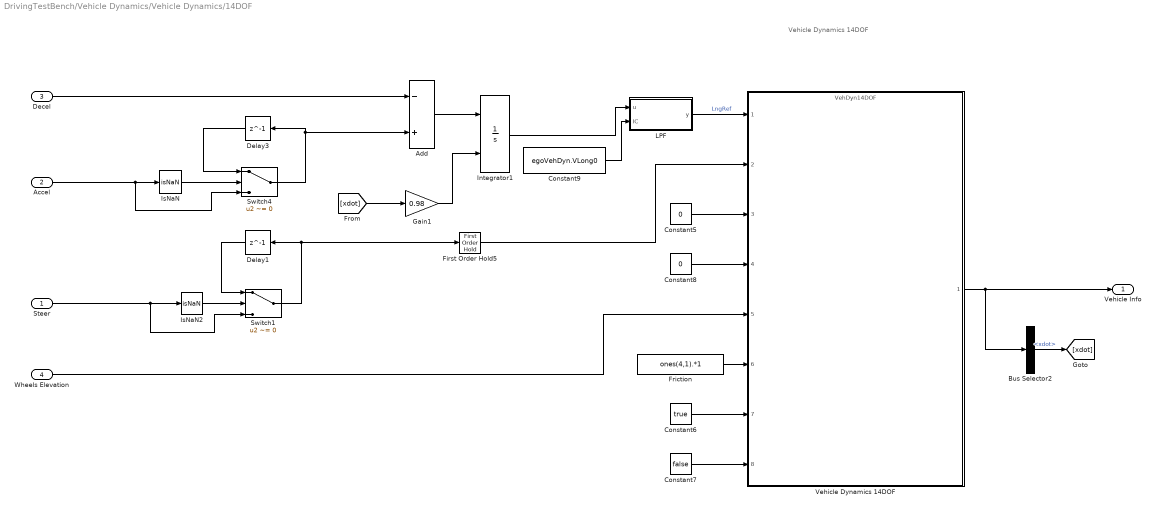
== system DrivingTestBench/Vehicle Dynamics/Vehicle Dynamics/14DOF ==
  note: Vehicle Dynamics 14DOF
  Steer : Inport
  Accel : Inport  Port=2
  Decel : Inport  Port=3
  Wheels Elevation : Inport  Port=4
  Add : Sum  Inputs=-+
  Bus Selector2 : BusSelector  OutputSignals=Body.BdyFrm.Cg.Vel.xdot
  Constant5 : Constant  Value=0
  Constant6 : Constant  Value=true  SampleTime=Ts
  Constant7 : Constant  Value=false
  Constant8 : Constant  Value=0
  Constant9 : Constant  Value=egoVehDyn.VLong0  SampleTime=Ts
  Delay1 : Delay  DelayLength=1
  Delay3 : Delay  DelayLength=1
  First Order Hold5 : FirstOrderHold  ErrorTolerance=.1  AllowContinuousInput=on
  Friction : Constant  Value=ones(4,1).*1  SampleTime=-1
  Gain1 : Gain  Gain=0.98
  Integrator1 : Integrator  InitialConditionSource=external  InitialCondition=egoVehDyn.VLong0  LimitOutput=on  UpperSaturationLimit=steadyStateSpeed-0.3  LowerSaturationLimit=eps
  IsNaN : RelationalOperator  Operator=isNaN  OutDataTypeStr=boolean  RndMeth=Simplest  InputSameDT=off
  IsNaN2 : RelationalOperator  Operator=isNaN  OutDataTypeStr=boolean  RndMeth=Simplest  InputSameDT=off
  LPF : Subsystem  mask{wc=2*pi}
      mask prompts: wc "Cut off frequency"
  Switch1 : Switch  Criteria=u2 ~= 0  SaturateOnIntegerOverflow=off  InputSameDT=off
  Switch4 : Switch  Criteria=u2 ~= 0  SaturateOnIntegerOverflow=off  InputSameDT=off
  Vehicle Dynamics 14DOF : ModelReference  ModelNameDialog=VehDyn14DOF.slx  UsingDefaultArgumentValue=0,0,0,0,0  SimulationMode=Normal  ModelReferenceVersion=10.0
  Vehicle Info : Outport
  wires:
  Decel/1 -> Add/1
  Vehicle Dynamics 14DOF/1 -> Vehicle Info/1, Bus Selector2/1
  Integrator1/1 -> LPF/1(u)
  Bus Selector2/1 -> [xdot]  "<xdot>"
  Constant7/1 -> Vehicle Dynamics 14DOF/8
  Constant5/1 -> Vehicle Dynamics 14DOF/3
  Constant8/1 -> Vehicle Dynamics 14DOF/4
  LPF/1(y) -> Vehicle Dynamics 14DOF/1  "LngRef"
  Constant9/1 -> LPF/2(IC)
  Gain1/1 -> Integrator1/2
  Constant6/1 -> Vehicle Dynamics 14DOF/7
  Friction/1 -> Vehicle Dynamics 14DOF/6
  Add/1 -> Integrator1/1
  Wheels Elevation/1 -> Vehicle Dynamics 14DOF/5
  First Order Hold5/1 -> Vehicle Dynamics 14DOF/2
  IsNaN/1 -> Switch4/2
  Accel/1 -> Switch4/3, IsNaN/1
  Switch4/1 -> Delay3/1, Add/2
  Delay3/1 -> Switch4/1
  Switch1/1 -> First Order Hold5/1, Delay1/1
  Delay1/1 -> Switch1/1
  IsNaN2/1 -> Switch1/2
  Steer/1 -> Switch1/3, IsNaN2/1
  [xdot] -> Gain1/1

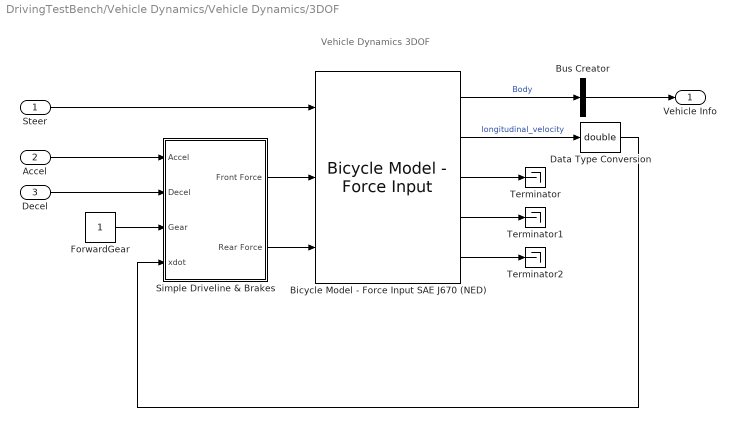
== system DrivingTestBench/Vehicle Dynamics/Vehicle Dynamics/3DOF ==
  note: Vehicle Dynamics 3DOF
  Steer : Inport
  Accel : Inport  Port=2
  Decel : Inport  Port=3
  Bicycle Model - Force Input SAE J670 (NED) : autolibshared/Bicycle Model - Force Input  trackMode=Single (bicycle)  inputMode=External longitudinal forces  frontSteerMode=on  rearSteerMode=off  windMode=off  muMode=off  extFMode=off  extMMode=off  aMode=3  NF=2  NR=2  m=egoVehDyn.Mass  a=egoVehDyn.CGToFrontAxle  b=egoVehDyn.CGToRearAxle  h=0.0375  X_o=egoVehDyn.X0  xdot_o=egoVehDyn.VLong0  CalphaMode=Constant  sigmaMode=on  w=[1.4,1.4]  Cy_f=12e3  Cy_r=11e3  sigma_f=.1  sigma_r=.1  alpha_f_brk=[-.1 .1]  Cy_f_data=[-9e3 9e3]  alpha_r_brk=[-.1 .1]  Cy_r_data=[-9e3 9e3]  Y_o=egoVehDyn.Y0  ydot_o=0  Izz=egoVehDyn.YawMomentOfInertia  psi_o=egoVehDyn.Yaw0  r_o=0  Af=0  Cd=.3  Cl=.1  Cpm=.1  beta_w=[0:0.01:0.3]  Cs=[0:0.03:0.9]  Cym=[0:0.01:0.3]  Pabs=101325  Tair=273  g=9.81  mu=1  xdot_tol=.01  Fznom=5000  Fxtire_sat=1e6  Fytire_sat=1e6  longOff=0  latOff=0  vertOff=0
      settings: LibrarySourceBlock=drivingscenarioandsensors/Bicycle Model - Force Input
      settings: AttributesFormatString=|
      | ---------------------------------
      | X_o = %<X_o>
      | Y_o = %<Y_o>
      | psi_o = %<psi_o>
      | xdot_o = %<xdot_o>
      | ydot_o = %<ydot_o>
  Bus Creator : BusCreator  Inputs=Body
  Data Type Conversion : DataTypeConversion  OutDataTypeStr=double  SaturateOnIntegerOverflow=off  RndMeth=Floor
  ForwardGear : Constant  SampleTime=Ts
  Simple Driveline & Brakes : Subsystem
  Terminator : Terminator
  Terminator1 : Terminator
  Terminator2 : Terminator
  Vehicle Info : Outport
  wires:
  Decel/1 -> Simple Driveline & Brakes/2(Decel)
  Accel/1 -> Simple Driveline & Brakes/1(Accel)
  Simple Driveline & Brakes/2(Rear Force) -> Bicycle Model - Force Input SAE J670 (NED)/3
  Bicycle Model - Force Input SAE J670 (NED)/2 -> Data Type Conversion/1  "longitudinal_velocity"
  ForwardGear/1 -> Simple Driveline & Brakes/3(Gear)
  Simple Driveline & Brakes/1(Front Force) -> Bicycle Model - Force Input SAE J670 (NED)/2
  Steer/1 -> Bicycle Model - Force Input SAE J670 (NED)/1
  Bicycle Model - Force Input SAE J670 (NED)/3 -> Terminator/1
  Data Type Conversion/1 -> Simple Driveline & Brakes/4(xdot)
  Bicycle Model - Force Input SAE J670 (NED)/1 -> Bus Creator/1  "Body"
  Bicycle Model - Force Input SAE J670 (NED)/4 -> Terminator1/1
  Bicycle Model - Force Input SAE J670 (NED)/5 -> Terminator2/1
  Bus Creator/1 -> Vehicle Info/1

== system DrivingTestBench/Scenario and Environment/Sensors/Lanes/No Lanes ==
  Ground : Ground
  Lanes : Outport  OutDataTypeStr=Bus: LaneBus
  wires:
  Ground/1 -> Lanes/1

== system DrivingTestBench/Scenario and Environment/Sensors/Lanes/Vision ==
  Ground Truth Lanes : roadrunnerscenario/RoadRunner Scenario Reader  TopicCategory=Sensor  ActorCategory=All Types  ActionType=Path Following  EventType=User-Defined  TopicType=Actor Specifications  VehicleType=Vehicle Specifications  TrafficSignalType=Traffic Signal Specifications  TrafficSignalControllerType=Traffic Signal Controller Specifications  UserDefinedAction=Action1  UserDefinedEvent=Event1  Filter=Self  AdditionalRelationship=None  SensorTopic=Lane Boundaries  LaneBoundaryOutputTopic=Ego-Lane  SensorID=3  SampleTime=Ts
  Message Receive1 : Receive  InputPortMessageModes=m  SampleTime=Ts
  Vision Detection Generator : drivingscenarioandsensors/Vision Detection Generator  SensorIndex=3  DetectorOutput=Lanes only  UpdateInterval=Ts  LaneUpdateInterval=0.01  SensorLocation=[cameraParams.Position(1), cameraParams.Position(2)]  Height=cameraParams.Position(3)  Yaw=cameraParams.Rotation(1)  Pitch=cameraParams.Rotation(2)  Roll=cameraParams.Rotation(3)  BusNameSource=Auto  BusName=BusVision  BusName2Source=Auto  BusName2=BusVisionLaneDetections1  MaxNumDetectionsSource=Property  MaxNumDetections=20  MaxNumLanesSource=Property  MaxNumLanes=2  DetectionCoordinates=Ego Cartesian  SimulateUsing=Code generation  MaxRange=cameraParams.DetectionRanges(2)-100  BoundingBoxAccuracy=5  ProcessNoiseIntensity=5  MaxSpeed=150  MaxAllowedOcclusion=0.5  MinObjectImageSize=[5 5]  DetectionProbability=0.9  FalsePositivesPerImage=0  MinLaneImageSize=[ 20, 5 ]  LaneBoundaryAccuracy=4  HasNoise=off  InitialSeedSource=Repeatable  InitialSeed=0  UsedSeed=driving.internal.SimulinkUtilities.seedManager(gcb)  ActorProfilesSource=MATLAB expression  ActorProfilesParameters=driving.internal.ActorProfilesParameters  ActorProfilesExpression=actorProfiles  Intrinsics=driving.internal.cameraIntrinsics(FocalLength=cameraParams.FocalLength,PrincipalPoint=cameraParams.PrincipalPoint,ImageSize=cameraParams.ImageSize)
  Lanes : Outport  OutDataTypeStr=Bus: LaneBus
  wires:
  Ground Truth Lanes/1 -> Message Receive1/1
  Message Receive1/1 -> Vision Detection Generator/1
  Vision Detection Generator/1 -> Lanes/1  "lane_detections"

== system DrivingTestBench/Scenario and Environment/Sensors/Object Detections/Camera and Radar ==
  note: Probabilistic Sensors
  Actors : Inport
  Time : Inport  Port=2
  Driving Radar Data Generator : drivingscenarioandsensors/Driving Radar Data Generator  Priority=-1  SensorIndex=2  UpdateRate=1/Ts  MountingLocation=radarParams.Position  MountingAngles=radarParams.Rotation  HasElevation=off  HasRangeRate=on  HasNoise=off  HasFalseAlarms=off  HasOcclusion=off  MaxNumReportsSource=Property  MaxNumReports=50  TargetReportFormat=Clustered detections  DetectionCoordinates=Body  TrackCoordinates=Body  BusNameSource=Auto  BusName=BusRadar  SimulateUsing=Interpreted execution  AzimuthResolution=radarParams.AzRes  ElevationResolution=5  RangeResolution=radarParams.RangeRes  RangeRateResolution=radarParams.RangeRateRes  AzimuthBiasFraction=0.05  ElevationBiasFraction=0.1  RangeBiasFraction=0.08  RangeRateBiasFraction=0.05  FieldOfView=radarParams.FieldOfView  RangeLimits=radarParams.DetectionRanges  RangeRateLimits=[ -100, 100 ]  DetectionProbability=0.99  FalseAlarmRate=1e-06  ReferenceRange=100  ReferenceRCS=0  CenterFrequency=77e9  FilterInitializationFcn=initcvekf  ConfirmationThreshold=[2 3]  DeletionThreshold=[5 5]  InitialSeedSource=Repeatable  InitialSeed=0  UsedSeed=matlabshared.tracking.internal.SimulinkUtilities.seedManager(gcb)  ProfilesSource=MATLAB expression  ProfilesParameters=driving.internal.ActorProfilesRadarParameters  ProfilesExpression=actorProfiles
  Sensor Fusion and Tracking : Subsystem
  Vision Detection Generator : drivingscenarioandsensors/Vision Detection Generator  Priority=-1  SensorIndex=1  DetectorOutput=Objects only  UpdateInterval=Ts  LaneUpdateInterval=Ts  SensorLocation=[cameraParams.Position(1), cameraParams.Position(2)]  Height=cameraParams.Position(3)  Yaw=cameraParams.Rotation(3)  Pitch=cameraParams.Rotation(2)  Roll=cameraParams.Rotation(1)  BusNameSource=Auto  BusName=BusVision  BusName2Source=Auto  BusName2=BusLaneDetections  MaxNumDetectionsSource=Property  MaxNumDetections=20  MaxNumLanesSource=Property  MaxNumLanes=30  DetectionCoordinates=Ego Cartesian  SimulateUsing=Interpreted execution  MaxRange=cameraParams.DetectionRanges(2)  BoundingBoxAccuracy=5  ProcessNoiseIntensity=5  MaxSpeed=50  MaxAllowedOcclusion=0.5  MinObjectImageSize=[ 15, 15 ]  DetectionProbability=0.99  FalsePositivesPerImage=0.001  MinLaneImageSize=[ 20, 5 ]  LaneBoundaryAccuracy=3  HasNoise=off  InitialSeedSource=Repeatable  InitialSeed=0  UsedSeed=driving.internal.SimulinkUtilities.seedManager(gcb)  ActorProfilesSource=MATLAB expression  ActorProfilesParameters=driving.internal.ActorProfilesParameters  ActorProfilesExpression=actorProfiles  Intrinsics=driving.internal.cameraIntrinsics(FocalLength=cameraParams.FocalLength,PrincipalPoint=cameraParams.PrincipalPoint,ImageSize=cameraParams.ImageSize)
  Tracks : Outport
  Camera Object Detections : Outport  Port=2
  wires:
  Time/1 -> Sensor Fusion and Tracking/1(System Time)
  Sensor Fusion and Tracking/1(Tracks) -> Tracks/1
  Driving Radar Data Generator/1 -> Sensor Fusion and Tracking/3(Radar)
  Vision Detection Generator/1 -> Camera Object Detections/1, Sensor Fusion and Tracking/2(Vision)
  Actors/1 -> Driving Radar Data Generator/1, Vision Detection Generator/1

== system DrivingTestBench/Scenario and Environment/Sensors/Object Detections/Ground Truth ==
  note: Ground Truth FOV Sensor
  Actors : Inport
  Time : Inport  Port=2
  Actors1 : InportShadow
  Ground Truth Camera : MATLABSystem  System=drivingApplication.internal.utils.IdealDetectionGenerator  SensorIndex=1  Sensor=cameraParams  SensorOutput=Object Detections  ActorProfiles=actorProfiles
      mask Type: drivingApplication.internal.utils.IdealDetectionGenerator
  Ground Truth Radar : MATLABSystem  System=drivingApplication.internal.utils.IdealDetectionGenerator  SensorIndex=2  Sensor=radarParams  SensorOutput=Tracks  ActorProfiles=actorProfiles
      mask Type: drivingApplication.internal.utils.IdealDetectionGenerator
  Time1 : InportShadow  Port=2
  Tracks : Outport
  Camera Object Detections : Outport  Port=2
  wires:
  Actors/1 -> Ground Truth Radar/1
  Ground Truth Radar/1 -> Tracks/1  "radar_truth_tracks"
  Time/1 -> Ground Truth Radar/2
  Time1/1 -> Ground Truth Camera/2
  Actors1/1 -> Ground Truth Camera/1
  Ground Truth Camera/1 -> Camera Object Detections/1  "camera_truth"

== system DrivingTestBench/Vehicle Dynamics/Vehicle Dynamics/14DOF/LPF ==
  u : Inport
  IC : Inport  Port=2
  Constant : Constant  Value=wc
  Divide : Product  Inputs=**
  Init : autolibutils/Cont LPF IC/Init  SystemSampleTime=-1  VariantActivationTime=update diagram  EmptyChoice=off  PassThrough=off  PassThroughVariantControl=(default)  EmptyChoiceVariantControl=(default)  AllowFlexibleInterface=on  Latency=0  AutoFrameSizeCalculation=off
  Integrator : Integrator  ExternalReset=rising  InitialConditionSource=external
  Sum : Sum  Inputs=|+-
  y : Outport  VectorParamsAs1DForOutWhenUnconnected=off
  wires:
  Integrator/1 -> y/1, Init/1
  IC/1 -> Init/2, Integrator/3
  u/1 -> Sum/1
  Init/1 -> Sum/2
  Constant/1 -> Divide/2
  Sum/1 -> Divide/1
  Divide/1 -> Integrator/1
  Init/2 -> Integrator/2

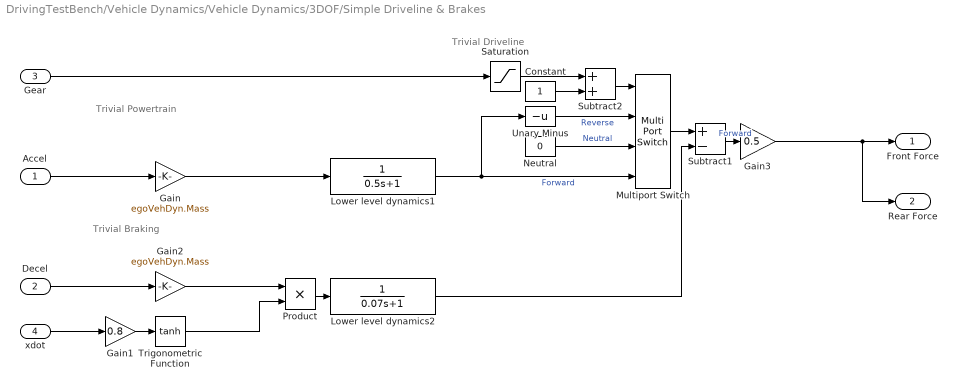
== system DrivingTestBench/Vehicle Dynamics/Vehicle Dynamics/3DOF/Simple Driveline & Brakes ==
  note: Trivial Driveline
  note: Trivial Powertrain
  note: Trivial Braking
  Accel : Inport
  Decel : Inport  Port=2
  Gear : Inport  Port=3
  xdot : Inport  Port=4
  Constant : Constant
  Gain : Gain  Gain=egoVehDyn.Mass
  Gain1 : Gain  Gain=0.8
  Gain2 : Gain  Gain=egoVehDyn.Mass
  Gain3 : Gain  Gain=0.5
  Lower level dynamics1 : TransferFcn  Denominator=[0.5 1]
  Lower level dynamics2 : TransferFcn  Denominator=[0.07 1]
  Multiport Switch : MultiPortSwitch  DataPortOrder=Zero-based contiguous  zeroidx=on  SaturateOnIntegerOverflow=off  InputSameDT=off
  Neutral : Constant  Value=0
  Product : Product
  Saturation : Saturate  UpperLimit=1  LowerLimit=-1  ZeroCross=off
  Subtract1 : Sum  Inputs=+-
  Subtract2 : Sum
  Trigonometric Function : Trigonometry  Operator=tanh
  Unary Minus : UnaryMinus
  Front Force : Outport  VectorParamsAs1DForOutWhenUnconnected=off
  Rear Force : Outport  Port=2  VectorParamsAs1DForOutWhenUnconnected=off
  wires:
  Multiport Switch/1 -> Subtract1/1
  Accel/1 -> Gain/1
  xdot/1 -> Gain1/1
  Decel/1 -> Gain2/1
  Trigonometric Function/1 -> Product/2
  Gain1/1 -> Trigonometric Function/1
  Gain/1 -> Lower level dynamics1/1
  Gain2/1 -> Product/1
  Lower level dynamics2/1 -> Subtract1/2
  Product/1 -> Lower level dynamics2/1
  Gear/1 -> Saturation/1
  Constant/1 -> Subtract2/2
  Subtract2/1 -> Multiport Switch/1
  Neutral/1 -> Multiport Switch/3  "Neutral"
  Lower level dynamics1/1 -> Unary Minus/1, Multiport Switch/4  "Forward"
  Saturation/1 -> Subtract2/1
  Subtract1/1 -> Gain3/1  "Forward"
  Unary Minus/1 -> Multiport Switch/2  "Reverse"
  Gain3/1 -> Front Force/1, Rear Force/1

== system DrivingTestBench/Scenario and Environment/Sensors/Object Detections/Camera and Radar/Sensor Fusion and Tracking ==
  note: Sensor Fusion
  System Time : Inport  OutDataTypeStr=double  PortDimensions=[1 1]  SampleTime=[Ts,0]  BusOutputAsStruct=on
  Vision : Inport  Port=2  OutDataTypeStr=Bus: BusVision  PortDimensions=[1 1]  SampleTime=[Ts,0]  BusOutputAsStruct=on
  Radar : Inport  Port=3  OutDataTypeStr=Bus: BusRadar  PortDimensions=[1 1]  SampleTime=[Ts,0]  BusOutputAsStruct=on
  Detection Concatenation : trackingutilitieslib/Detection Concatenation  NumInputs=2  BusNameSource=Auto  BusName=BusDetectionConcatenation  SimulateUsing=Code generation
  Multi-Object Tracker : drivinglib/Multi-Object Tracker  TrackerIndex=uint32( 0 )  FilterInitializationFcn=initcvekf  AssignmentThreshold=trackingParams.assigThresh  ConfirmationThreshold=[trackingParams.M,trackingParams.N]  DeletionThreshold=[trackingParams.numCoasts,trackingParams.numCoasts]  MaxNumTracks=trackingParams.numTracks  MaxNumSensors=trackingParams.numSensors  OOSMHandling=Terminate  StateParametersSimulink=struct  HasStateParametersInput=off  TimeInputSource=Input port  HasCostMatrixInput=off  HasDetectableTrackIDsInput=off  BusNameSource=Auto  BusName=BusMultiObjectTracker1  TentativeTracksOutputPort=off  AllTracksOutputPort=off  SimulateUsing=Code generation
  Tracks : Outport  OutDataTypeStr=Bus: BusMultiObjectTracker1  PortDimensions=[1 1]  SampleTime=[Ts,0]  VectorParamsAs1DForOutWhenUnconnected=off  BusOutputAsStruct=on
  wires:
  Radar/1 -> Detection Concatenation/2
  Detection Concatenation/1 -> Multi-Object Tracker/1
  Multi-Object Tracker/1 -> Tracks/1
  Vision/1 -> Detection Concatenation/1
  System Time/1 -> Multi-Object Tracker/2

== matlab function DrivingTestBench/Scenario and Environment/Test Enable/Pack Lane Detections/MATLAB Function ==
  data: laterOffset input; strengthOut output; strength input
function strengthOut = fcn(laterOffset,strength)

if isnan(laterOffset)
    strengthOut = 0;
else
    strengthOut = strength;
end

== matlab function DrivingTestBench/Scenario and Environment/Test Enable/Pack Lane Detections/MATLAB Function1 ==
  data: laterOffset input; strengthOut output; strength input
function strengthOut = fcn(laterOffset,strength)

if isnan(laterOffset)
    strengthOut = 0;
else
    strengthOut = strength;
end

== matlab function DrivingTestBench/Scenario and Environment/Test Enable/Calculate DTLE ==
  data: laneDetections input; actorPose input; leftDTLE output; actorProfiles parameter; rightDTLE output; isOutOfLane output; dtleThreshold parameter; egoActorID parameter
function [leftDTLE, rightDTLE, isOutOfLane] = calculateDTLE(laneDetections, actorPose, actorProfiles, dtleThreshold, egoActorID)
    % Calculate the Distance to Lane Edge (DTLE) using clothoid lane boundaries
    % and visualize the results

% Initialize outputs
wheelbase = 0;
trackWidth = 0;

% Extract the number of actors
numActors = length(actorProfiles);

% Initialize an array to store ActorIDs
actorIDs = zeros(1, numActors);

% Extract ActorIDs using a loop for code generation compatibility
for i = 1:numActors
    actorIDs(i) = actorProfiles(i).ActorID;
end

% Find the index of the ego actor
egoIndexinActorProfile = find(actorIDs == egoActorID, 1);

% Check if the ego actor index is valid
if ~isempty(egoIndexinActorProfile)
    % Extract the entire ego actor struct
    egoActor = actorProfiles(egoIndexinActorProfile);
    
    % Extract vehicle dimensions
    lengthValue = egoActor.Length;
    frontOverhang = egoActor.FrontOverhang;
    rearOverhang = egoActor.RearOverhang;
    widthValue = egoActor.Width;
    
    % Calculate wheelbase and track width
    wheelbase = lengthValue - (frontOverhang + rearOverhang);
    trackWidth = estimateTrackWidth(widthValue);
end
    % Extract vehicle dimensions
    % wheelbase = actorProfiles(egoIndexinActorProfile).Length - (actorProfiles(egoIndexinActorProfile).FrontOverhang + actorProfiles(egoIndexinActorProfile).RearOverhang);
    % trackWidth = estimateTrackWidth(actorProfiles, egoIndexinActorProfile);

    % Ensure input types are consistent
    vehiclePos = single(actorPose.Position(1:2)); % Use both x and y for 2D calculation
    vehicleYaw = deg2rad(single(actorPose.Yaw));  % Convert yaw from degrees to radians

    % Calculate the position of the front axle in the global coordinate system
    frontAxlePos = vehiclePos + [wheelbase/2 * cos(vehicleYaw), wheelbase/2 * sin(vehicleYaw)];

    % Calculate the position of the front tires
    frontLeftTire = frontAxlePos + [-trackWidth/2 * sin(vehicleYaw), trackWidth/2 * cos(vehicleYaw)];
    frontRightTire = frontAxlePos + [trackWidth/2 * sin(vehicleYaw), -trackWidth/2 * cos(vehicleYaw)];

    % Initialize DTLE values as single
    leftDTLE = single(inf);
    rightDTLE = single(inf);

    % Check the left lane boundary
    if ~isnan(laneDetections.Left.LateralOffset)
        leftDTLE = single(laneDetections.Left.LateralOffset) - (vehiclePos(2) - single(frontLeftTire(2)));
    end

    % Check the right lane boundary
    if ~isnan(laneDetections.Right.LateralOffset)
        % Correct the calculation for the right DTLE
        rightDTLE = (vehiclePos(2) - single(frontRightTire(2))) - single(laneDetections.Right.LateralOffset);
    end

    % Determine if the vehicle is going out of the lane
    isOutOfLane = (leftDTLE <= dtleThreshold) || (rightDTLE <= dtleThreshold);
end


function trackWidth = estimateTrackWidth(egoActorWidth)
% estimateTrackWidth estimates the track width from egoActorWidth information.
%

% Assumption: The wheels are symmetrically placed about the centerline of the vehicle.
% Calculate the estimated track width as a proportion of the overall width.
% This proportion can vary based on vehicle type; here, we use a typical value.
bodyOverhang = 0.2678; % Body overhang value (in meters) from the edge to the wheel center
trackWidth = egoActorWidth - 2 * bodyOverhang;
end

== matlab function DrivingTestBench/Scenario and Environment/Test Enable/Test Start Enable ==
  data: testEnable output; testStartPosition input; currentPosition input
function testEnable = testStartEnable(testStartPosition, currentPosition)

persistent previousError;
if(isempty(previousError))
    previousError = inf;
end

currentError = norm(testStartPosition-currentPosition);

if(currentError>=previousError && previousError~=inf)
    testEnable = true;
else
    testEnable = false;
end

previousError = currentError;

end

== matlab function DrivingTestBench/Scenario and Environment/Test Enable/Ego Speed ==
  data: speed output; velocity input
function speed = egoSpeed(velocity)

speed = norm([velocity(1), velocity(2), velocity(3)]);

== matlab function DrivingTestBench/Scenario and Environment/RR Simulation Stop ==
  data: stop input boolean
function simStop(stop)

coder.extrinsic('configureDrivingTestBench.stopSimulation');
configureDrivingTestBench.stopSimulation(stop)

end

== matlab function DrivingTestBench/Scenario and Environment/Filter Tracks ==
  data: testEnable input boolean; inpTracks input; tracks output Bus: BusMultiObjectTracker1
function tracks = filterTracks(testEnable, inpTracks)

tracks = inpTracks;

% Filter tracks if test is not enabled.
if(testEnable==0)
    tracks.NumTracks = 0;
end

end
